simulink model "dcm_flyback_avg_model_student_2019a(1)"  (R2019a)
settings: Solver=ode23tb  StartTime=0.0  StopTime=.8  MaxStep=(1/60)/1000  RelTol=1e-6
undefined symbols (not defined in the file): C, Cf, duty, fL, Lf, Lm, n1, np, Ts, Vgrms
libraries: powerlib x23, powerlib_meascontrol x1
settings Model: Creator=jvr2131  LastModifiedBy=john
settings SolverCC: AlgebraicLoopSolver=LineSearch
settings DataIOCC: LimitDataPoints=on  SaveFormat=Array  ReturnWorkspaceOutputs=off
settings OptimizationCC: BlockReduction=off  BooleanDataType=off  LifeSpan=inf
settings DebuggingCC: SaveWithParameterizedLinksMsg=none  UnderspecifiedInitializationDetection=Classic  MergeDetectMultiDrivingBlocksExec=none  SignalResolutionControl=TryResolveAllWithWarning  MultiTaskDSMMsg=warning  MultiTaskCondExecSysMsg=none  StateNameClashWarn=warning  SFUnexpectedBacktrackingDiag=warning  SFNoUnconditionalDefaultTransitionDiag=warning  SFExecutionAtInitializationDiag=none  ArithmeticOperatorsInVariantConditions=warning
settings HardwareCC: ProdBitPerPointer=32  ProdBitPerSizeT=32  ProdBitPerPtrDiffT=32  ProdLargestAtomicFloat=None  ProdIntDivRoundTo=Undefined  ProdEndianess=Unspecified  ProdWordSize=32  ProdHWDeviceType=32-bit Generic  TargetUnknown=on
settings ModelReferenceCC: PropagateSignalLabelsOutOfModel=off
settings SFSimCC: SimUseLocalCustomCode=off
settings RTWCC: RTWUseLocalCustomCode=off
settings CodeAppCC: StateflowObjectComments=on
settings GRTTargetCC: TargetLangStandard=C89/C90 (ANSI)  GeneratePreprocessorConditionals=Disable all
settings ConfigComp: CovMetricSettings=dw  CovHtmlReporting=on  CovSaveCumulativeToWorkspaceVar=on  CovSaveSingleToWorkspaceVar=on  CovExternalEMLEnable=off
settings SimscapeCC: SimscapeNormalizeSystem=off

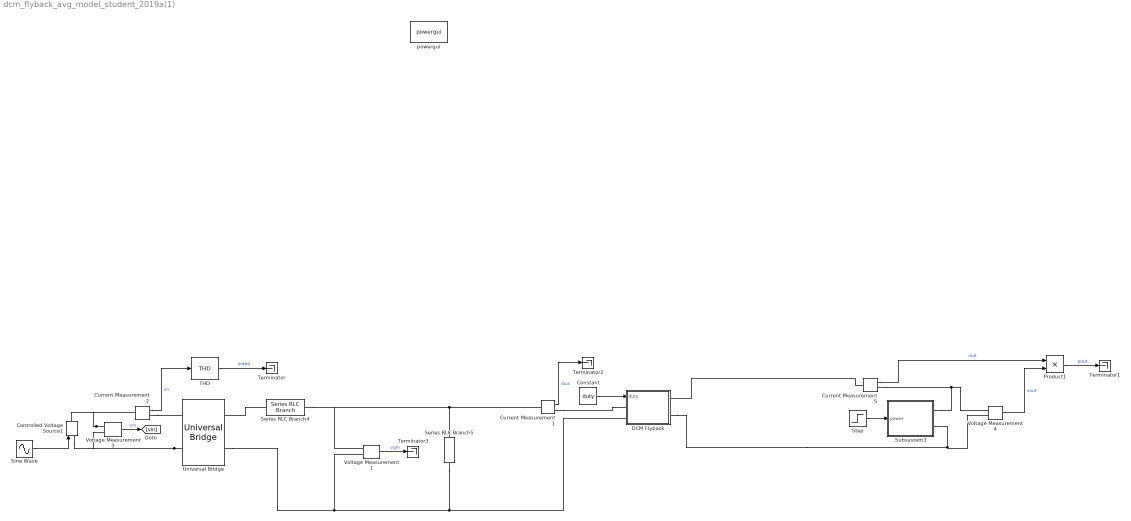
== system dcm_flyback_avg_model_student_2019a(1) ==
  Constant : Constant  Value=duty
  Controlled Voltage Source1 : powerlib/Electrical Sources/Controlled Voltage Source  Initialize=on  Source_Type=AC  Amplitude=0  Phase=0  Frequency=0  Measurements=None
      settings: SourceProductName=Simscape Electrical
  Current Measurement1 : powerlib/Measurements/Current Measurement  PhasorSimulation=off  OutputType=Complex  PSBequivalent=0
      settings: SourceProductName=Simscape Electrical
  Current Measurement2 : powerlib/Measurements/Current Measurement  PhasorSimulation=off  OutputType=Complex  PSBequivalent=0
      settings: SourceProductName=Simscape Electrical
  Current Measurement5 : powerlib/Measurements/Current Measurement  PhasorSimulation=off  OutputType=Complex  PSBequivalent=0
      settings: SourceProductName=Simscape Electrical
  DCM Flyback : Subsystem  mask{np=np, n1=n1, Lm=Lm, C=C, Ts=Ts}
      mask prompts: np "Primary Turns"; n1 "Secondary Turns"; Lm "Mag Inductance (primary)"; C "Output Capacitance"; Ts "Switching Period"
  Product1 : Product
  Series RLC Branch4 : powerlib/Elements/Series RLC Branch  LConnTagsString=__new0  RConnTagsString=__new0  BranchType=L  Resistance=1  Inductance=Lf  SetiL0=off  InitialCurrent=0  Capacitance=C  Setx0=on  InitialVoltage=V  Measurements=None
      settings: SourceProductName=Simscape Electrical
  Series RLC Branch5 : powerlib/Elements/Series RLC Branch  LConnTagsString=__new0  RConnTagsString=__new0  BranchType=C  Resistance=1  Inductance=1e-3  SetiL0=off  InitialCurrent=0  Capacitance=Cf  Setx0=off  InitialVoltage=V  Measurements=None
      settings: SourceProductName=Simscape Electrical
  Sine Wave : Sin  Amplitude=Vgrms*sqrt(2)  Frequency=2*pi*fL  SampleTime=0
  Step : Step  Time=0  Before=power  After=power  SampleTime=0
  Subsystem3 : Subsystem
  THD : powerlib_meascontrol/Measurements/THD  Freq=fL  Ts=0
      settings: SourceProductName=Simscape Electrical
  Terminator{,1..3} (4 alike) : Terminator
  Universal Bridge : powerlib/Power Electronics/Universal Bridge  Arms=2  SnubberResistance=1e5  SnubberCapacitance=inf  Device=Diodes  Ron=.1e-3  Lon=0  ForwardVoltages="[  0  0  ]"  ForwardVoltage=0  GTOparameters=[ 10e-6 , 20e-6 ]  IGBTparameters=[ 1e-6 , 2e-6 ]  Measurements=None  Measurements_2=None  converterType=Rectifier
      settings: SourceProductName=Simscape Electrical
  Voltage Measurement1 : powerlib/Measurements/Voltage Measurement  PhasorSimulation=off  OutputType=Complex  PSBequivalent=0
      settings: SourceProductName=Simscape Electrical
  Voltage Measurement3 : powerlib/Measurements/Voltage Measurement  PhasorSimulation=off  OutputType=Complex  PSBequivalent=0
      settings: SourceProductName=Simscape Electrical
  Voltage Measurement4 : powerlib/Measurements/Voltage Measurement  PhasorSimulation=off  OutputType=Complex  PSBequivalent=0
      settings: SourceProductName=Simscape Electrical
  powergui : powerlib/powergui  Priority=1  SimulationMode=Continuous  SampleTime=Ts/1000  frequency=60  Iterations=50  frequencyindice=0  Pbase=100e6  ErrMax=1e-4  UnitsV=kV  UnitsW=MW  buscounter=0  FunctionMessages=off  echomessages=off  EnableUseOfTLC=off  CurrentSourceSwitches=off  DisableSnubberDevices=off  DisableRonSwitches=off  DisableVfSwitches=off  DisplayEquations=off  AutomaticDiscreteSolvers=off  SolverType=Tustin/Backward Euler (TBE)  Interpol=off  ExternalGateDelay=off  methode=off  Ts=100  x0status=blocks  SPID=on  SwTol=0  HookPort=off  NonlinearTolerance=1e-4  nMaxIteration=100  ContinueOnMaxIteration=off  RestoreLinks=warning  ResistiveCurrentMeasurement=off  Frange=[0:2:500]  Ylog=off  Xlog=on  ShowGrid=off  save=off  variable=ZData  structure=0  ZoomFFT=off  StartTime=0.0  cycles=1  DisplayStyle=1  fundamental=60  FreqAxis=off  MaxFrequency=1000  frequencyindicesteady=1  RmsSteady=1  display=off
      settings: SourceProductName=Simscape Electrical
  wires:
  Voltage Measurement3/1 -> [vin]  "vin"
  Sine Wave/1 -> Controlled Voltage Source1/1
  Current Measurement2/1 -> THD/1  "iin"
  THD/1 -> Terminator/1  "iinthd"
  Voltage Measurement4/1 -> Product1/2  "vout"
  Current Measurement1/1 -> Terminator2/1  "ibus"
  Current Measurement5/1 -> Product1/1  "iout"
  Product1/1 -> Terminator1/1  "pout"
  Step/1 -> Subsystem3/1(power)
  Voltage Measurement1/1 -> Terminator3/1  "vgin"
  Constant/1 -> DCM Flyback/1(duty)
  connections:
  Universal Bridge/LConn2 -- Voltage Measurement3/LConn2 -- Controlled Voltage Source1/LConn1
  Voltage Measurement3/LConn1 -- Current Measurement2/LConn1 -- Controlled Voltage Source1/RConn1
  Current Measurement2/RConn1 -- Universal Bridge/LConn1
  Universal Bridge/RConn2 -- Series RLC Branch5/RConn1 -- DCM Flyback/LConn2 -- Voltage Measurement1/LConn2
  Subsystem3/RConn1 -- Current Measurement5/RConn1 -- Voltage Measurement4/LConn1
  Current Measurement1/RConn1 -- DCM Flyback/LConn1
  Current Measurement5/LConn1 -- DCM Flyback/RConn1
  Current Measurement1/LConn1 -- Series RLC Branch4/RConn1 -- Voltage Measurement1/LConn1 -- Series RLC Branch5/LConn1
  Series RLC Branch4/LConn1 -- Universal Bridge/RConn1
  Voltage Measurement4/LConn2 -- DCM Flyback/RConn2 -- Subsystem3/RConn2

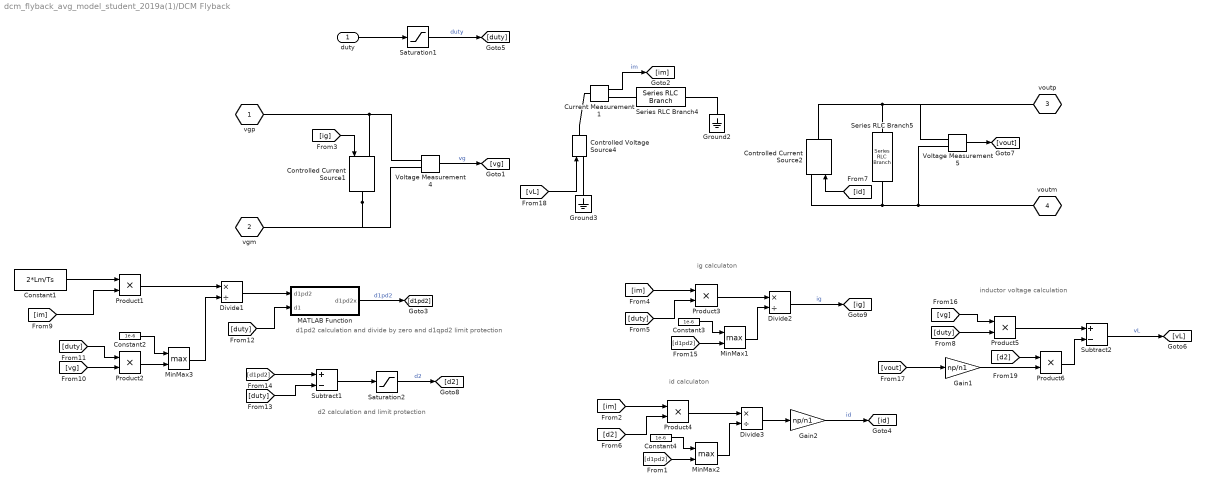
== system dcm_flyback_avg_model_student_2019a(1)/DCM Flyback ==
  note: inductor voltage calculation
  note: ig calculaton
  note: d2 calculation and limit protection
  note: d1pd2 calculation and divide by zero and d1qpd2 limit protection
  note: id calculaton
  duty : Inport
  Constant1 : Constant  Value=2*Lm/Ts
  Constant2 : Constant  Value=1e-6
  Constant3 : Constant  Value=1e-6
  Constant4 : Constant  Value=1e-6
  Controlled Current Source1 : powerlib/Electrical Sources/Controlled Current Source  Initialize=on  Source_Type=AC  Amplitude=0  Phase=0  Frequency=0  Measurements=None
      settings: SourceProductName=Simscape Electrical
  Controlled Current Source2 : powerlib/Electrical Sources/Controlled Current Source  Initialize=on  Source_Type=AC  Amplitude=0  Phase=0  Frequency=0  Measurements=None
      settings: SourceProductName=Simscape Electrical
  Controlled Voltage Source4 : powerlib/Electrical Sources/Controlled Voltage Source  Initialize=on  Source_Type=AC  Amplitude=0  Phase=0  Frequency=0  Measurements=None
      settings: SourceProductName=Simscape Electrical
  Current Measurement1 : powerlib/Measurements/Current Measurement  PhasorSimulation=off  OutputType=Complex  PSBequivalent=0
      settings: SourceProductName=Simscape Electrical
  Divide1 : Product  Inputs=*/
  Divide2 : Product  Inputs=*/
  Divide3 : Product  Inputs=*/
  Gain1 : Gain  Gain=np/n1
  Gain2 : Gain  Gain=np/n1
  Ground2 : powerlib/Elements/Ground  LConnTagsString=a
      settings: SourceProductName=Simscape Electrical
  Ground3 : powerlib/Elements/Ground  LConnTagsString=a
      settings: SourceProductName=Simscape Electrical
  MATLAB Function : MATLAB Function  TreatAsAtomicUnit=on
  MinMax1 : MinMax  Function=max  Inputs=2
  MinMax2 : MinMax  Function=max  Inputs=2
  MinMax3 : MinMax  Function=max  Inputs=2
  Product{1..6} (6 alike) : Product
  Saturation1 : Saturate  UpperLimit=1  LowerLimit=0
  Saturation2 : Saturate  UpperLimit=1  LowerLimit=0
  Series RLC Branch4 : powerlib/Elements/Series RLC Branch  LConnTagsString=__new0  RConnTagsString=__new0  BranchType=L  Resistance=1  Inductance=Lm  SetiL0=off  InitialCurrent=0  Capacitance=C  Setx0=on  InitialVoltage=V  Measurements=None
      settings: SourceProductName=Simscape Electrical
  Series RLC Branch5 : powerlib/Elements/Series RLC Branch  LConnTagsString=__new0  RConnTagsString=__new0  BranchType=C  Resistance=1  Inductance=1e-3  SetiL0=off  InitialCurrent=0  Capacitance=C  Setx0=on  InitialVoltage=V  Measurements=None
      settings: SourceProductName=Simscape Electrical
  Subtract1 : Sum  Inputs=+-
  Subtract2 : Sum  Inputs=+-
  Voltage Measurement4 : powerlib/Measurements/Voltage Measurement  PhasorSimulation=off  OutputType=Complex  PSBequivalent=0
      settings: SourceProductName=Simscape Electrical
  Voltage Measurement5 : powerlib/Measurements/Voltage Measurement  PhasorSimulation=off  OutputType=Complex  PSBequivalent=0
      settings: SourceProductName=Simscape Electrical
  vgp : PMIOPort  Tag=PMCPort  Side=Left
  vgm : PMIOPort  Tag=PMCPort  Port=2  Side=Left
  voutp : PMIOPort  Tag=PMCPort  Port=3  Side=Right
  voutm : PMIOPort  Tag=PMCPort  Port=4  Side=Right
  wires:
  Current Measurement1/1 -> [im]  "im"
  Voltage Measurement5/1 -> [vout]
  duty/1 -> Saturation1/1
  [ig] -> Controlled Current Source1/1
  Voltage Measurement4/1 -> [vg]  "vg"
  Saturation1/1 -> [duty]  "duty"
  Constant1/1 -> Product1/1
  [im] -> Product1/2
  [vg] -> Product2/2
  [duty] -> Product2/1
  Product1/1 -> Divide1/1
  Product2/1 -> MinMax3/2
  MinMax3/1 -> Divide1/2
  Constant2/1 -> MinMax3/1
  [duty] -> MATLAB Function/2(d1)
  Divide1/1 -> MATLAB Function/1(d1pd2)
  MATLAB Function/1(d1pd2x) -> [d1pd2]  "d1pd2"
  [d1pd2] -> Subtract1/1
  [duty] -> Subtract1/2
  Subtract1/1 -> Saturation2/1
  Saturation2/1 -> [d2]  "d2"
  [im] -> Product3/1
  [duty] -> Product3/2
  Product3/1 -> Divide2/1
  [d1pd2] -> MinMax1/2
  MinMax1/1 -> Divide2/2
  Constant3/1 -> MinMax1/1
  Divide2/1 -> [ig]  "ig"
  [d1pd2] -> MinMax2/2
  [d2] -> Product4/2
  MinMax2/1 -> Divide3/2
  Product4/1 -> Divide3/1
  [im] -> Product4/1
  Constant4/1 -> MinMax2/1
  Divide3/1 -> Gain2/1
  Gain2/1 -> [id]  "id"
  [id] -> Controlled Current Source2/1
  [duty] -> Product5/2
  [vg] -> Product5/1
  Product5/1 -> Subtract2/1
  [vout] -> Gain1/1
  Gain1/1 -> Product6/2
  Product6/1 -> Subtract2/2
  Subtract2/1 -> [vL]  "vL"
  [vL] -> Controlled Voltage Source4/1
  [d2] -> Product6/1
  connections:
  Voltage Measurement5/LConn2 -- voutm/RConn1 -- Series RLC Branch5/RConn1 -- Controlled Current Source2/LConn1
  Controlled Current Source1/LConn1 -- vgp/RConn1 -- Voltage Measurement4/LConn1
  Controlled Current Source1/RConn1 -- vgm/RConn1 -- Voltage Measurement4/LConn2
  Ground3/LConn1 -- Controlled Voltage Source4/LConn1
  Current Measurement1/RConn1 -- Series RLC Branch4/LConn1
  Controlled Current Source2/RConn1 -- voutp/RConn1 -- Voltage Measurement5/LConn1 -- Series RLC Branch5/LConn1
  Ground2/LConn1 -- Series RLC Branch4/RConn1
  Controlled Voltage Source4/RConn1 -- Current Measurement1/LConn1

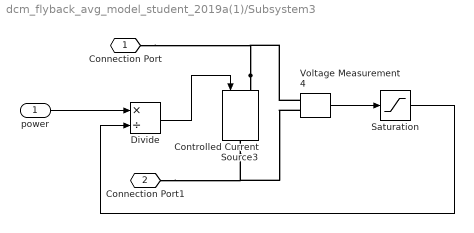
== system dcm_flyback_avg_model_student_2019a(1)/Subsystem3 ==
  power : Inport
  Controlled Current Source3 : powerlib/Electrical Sources/Controlled Current Source  Initialize=on  Source_Type=AC  Amplitude=0  Phase=0  Frequency=0  Measurements=None
      settings: SourceProductName=Simscape Electrical
  Divide : Product  Inputs=*/
  Saturation : Saturate  UpperLimit=inf  LowerLimit=1e-3
  Voltage Measurement4 : powerlib/Measurements/Voltage Measurement  PhasorSimulation=off  OutputType=Complex  PSBequivalent=0
      settings: SourceProductName=Simscape Electrical
  Connection Port : PMIOPort  Side=Right
  Connection Port1 : PMIOPort  Port=2  Side=Right
  wires:
  Saturation/1 -> Divide/2
  power/1 -> Divide/1
  Voltage Measurement4/1 -> Saturation/1
  Divide/1 -> Controlled Current Source3/1
  connections:
  Controlled Current Source3/RConn1 -- Connection Port1/RConn1 -- Voltage Measurement4/LConn2
  Controlled Current Source3/LConn1 -- Connection Port/RConn1 -- Voltage Measurement4/LConn1

== matlab function dcm_flyback_avg_model_student_2019a(1)/DCM Flyback/MATLAB Function ==
  data: d1pd2 input; d1pd2x output; d1 input
function d1pd2x = fcn(d1pd2,d1)

d1pd2x = d1pd2;

if(d1pd2<=d1)
    d1pd2=d1;
end

if(d1pd2>=1)
    d1pd2=1;
end

end
